simulink library "threeTetCtrllr_ul"  (R2018b)
settings: Solver=VariableStepAuto  StartTime=0.0  StopTime=10.0  RelTol=1e-3
values from neighbouring files (symbols this model uses):
  ctrl = CTR.threeThrCtlr    [threeTetCtrllr_ts.m]
libraries: filteredPIDController_ul x6
settings Model: Creator=Ayaz  LastModifiedBy=asiddiq2

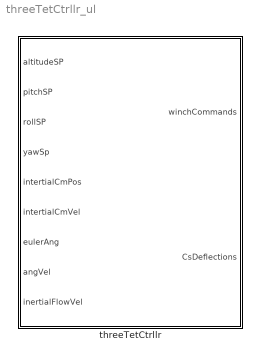
== system threeTetCtrllr_ul ==
  threeTetCtrllr : Subsystem

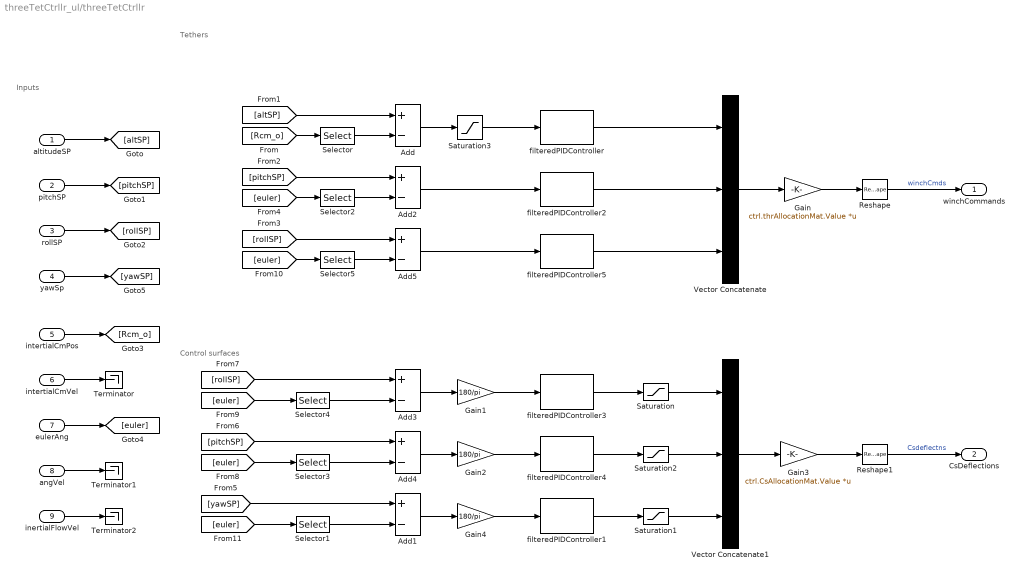
== system threeTetCtrllr_ul/threeTetCtrllr ==
  note: Inputs
  note: Control surfaces
  note: Tethers
  altitudeSP : Inport
  pitchSP : Inport  Port=2
  rollSP : Inport  Port=3
  yawSp : Inport  Port=4
  intertialCmPos : Inport  Port=5
  intertialCmVel : Inport  Port=6
  eulerAng : Inport  Port=7
  angVel : Inport  Port=8
  inertialFlowVel : Inport  Port=9
  Add{,1..5} (6 alike) : Sum  Inputs=+-
  Gain : Gain  Gain=ctrl.thrAllocationMat.Value  Multiplication=Matrix(K*u)
  Gain1 : Gain  Gain=180/pi
  Gain2 : Gain  Gain=180/pi
  Gain3 : Gain  Gain=ctrl.CsAllocationMat.Value  Multiplication=Matrix(K*u)
  Gain4 : Gain  Gain=180/pi
  Reshape : Reshape  OutputDimensionality=Row vector (2-D)
  Reshape1 : Reshape  OutputDimensionality=Column vector (2-D)
  Saturation : Saturate  UpperLimit=ctrl.aileronMaxDef.Value  LowerLimit=-ctrl.aileronMaxDef.Value
  Saturation1 : Saturate  UpperLimit=ctrl.rudderMaxDef.Value  LowerLimit=-ctrl.rudderMaxDef.Value
  Saturation2 : Saturate  UpperLimit=ctrl.elevatorMaxDef.Value  LowerLimit=-ctrl.elevatorMaxDef.Value
  Saturation3 : Saturate  UpperLimit=ctrl.altiErrorSat.Value  LowerLimit=-ctrl.altiErrorSat.Value
  Selector : Selector  NumberOfDimensions=2  InputPortWidth=3  IndexOptions=Index vector (dialog),Index vector (dialog)  Indices=3,1  OutputSizes=1,1
  Selector1 : Selector  NumberOfDimensions=2  InputPortWidth=3  IndexOptions=Index vector (dialog),Index vector (dialog)  Indices=1,1  OutputSizes=1,1
  Selector2 : Selector  NumberOfDimensions=2  InputPortWidth=3  IndexOptions=Index vector (dialog),Index vector (dialog)  Indices=2,1  OutputSizes=1,1
  Selector3 : Selector  NumberOfDimensions=2  InputPortWidth=3  IndexOptions=Index vector (dialog),Index vector (dialog)  Indices=2,1  OutputSizes=1,1
  Selector4 : Selector  NumberOfDimensions=2  InputPortWidth=3  IndexOptions=Index vector (dialog),Index vector (dialog)  Indices=1,1  OutputSizes=1,1
  Selector5 : Selector  NumberOfDimensions=2  InputPortWidth=3  IndexOptions=Index vector (dialog),Index vector (dialog)  Indices=1,1  OutputSizes=1,1
  Terminator : Terminator
  Terminator1 : Terminator
  Terminator2 : Terminator
  Vector Concatenate : Concatenate  NumInputs=3
  Vector Concatenate1 : Concatenate  NumInputs=3
  filteredPIDController : filteredPIDController_ul/filteredPIDController  kp=ctrl.altiTetherKp.Value  ki=ctrl.altiTetherKi.Value  kd=ctrl.altiTetherKd.Value  Value=ctrl.altiTetherTau.Value
  filteredPIDController1 : filteredPIDController_ul/filteredPIDController  kp=ctrl.rudderKp.Value  ki=ctrl.rudderKi.Value  kd=ctrl.rudderKd.Value  Value=ctrl.rudderTau.Value
  filteredPIDController2 : filteredPIDController_ul/filteredPIDController  kp=ctrl.pitchTetherKp.Value  ki=ctrl.pitchTetherKi.Value  kd=ctrl.pitchTetherKd.Value  Value=ctrl.pitchTetherTau.Value
  filteredPIDController3 : filteredPIDController_ul/filteredPIDController  kp=ctrl.aileronKp.Value  ki=ctrl.aileronKi.Value  kd=ctrl.aileronKd.Value  Value=ctrl.aileronTau.Value
  filteredPIDController4 : filteredPIDController_ul/filteredPIDController  kp=ctrl.elevatorKp.Value  ki=ctrl.elevatorKi.Value  kd=ctrl.elevatorKd.Value  Value=ctrl.elevatorTau.Value
  filteredPIDController5 : filteredPIDController_ul/filteredPIDController  kp=ctrl.rollTetherKp.Value  ki=ctrl.rollTetherKi.Value  kd=ctrl.rollTetherKd.Value  Value=ctrl.rollTetherTau.Value
  winchCommands : Outport
  CsDeflections : Outport  Port=2
  wires:
  Add3/1 -> Gain1/1
  Add4/1 -> Gain2/1
  filteredPIDController3/1 -> Saturation/1
  filteredPIDController4/1 -> Saturation2/1
  Selector3/1 -> Add4/2
  [euler] -> Selector3/1
  [pitchSP] -> Add4/1
  Selector4/1 -> Add3/2
  [euler] -> Selector4/1
  Saturation/1 -> Vector Concatenate1/1
  Vector Concatenate1/1 -> Gain3/1
  altitudeSP/1 -> [altSP]
  pitchSP/1 -> [pitchSP]
  rollSP/1 -> [rollSP]
  intertialCmPos/1 -> [Rcm_o]
  eulerAng/1 -> [euler]
  intertialCmVel/1 -> Terminator/1
  angVel/1 -> Terminator1/1
  inertialFlowVel/1 -> Terminator2/1
  Reshape1/1 -> CsDeflections/1  "Csdeflectns"
  Gain1/1 -> filteredPIDController3/1
  Gain2/1 -> filteredPIDController4/1
  [rollSP] -> Add3/1
  Gain4/1 -> filteredPIDController1/1
  [euler] -> Selector1/1
  Selector1/1 -> Add1/2
  [yawSP] -> Add1/1
  filteredPIDController1/1 -> Saturation1/1
  Add1/1 -> Gain4/1
  Selector/1 -> Add/2
  filteredPIDController2/1 -> Vector Concatenate/2
  Saturation3/1 -> filteredPIDController/1
  filteredPIDController5/1 -> Vector Concatenate/3
  Add5/1 -> filteredPIDController5/1
  Add2/1 -> filteredPIDController2/1
  filteredPIDController/1 -> Vector Concatenate/1
  Vector Concatenate/1 -> Gain/1
  Selector5/1 -> Add5/2
  Add/1 -> Saturation3/1
  Selector2/1 -> Add2/2
  Gain/1 -> Reshape/1
  Saturation1/1 -> Vector Concatenate1/3
  Reshape/1 -> winchCommands/1  "winchCmds"
  [altSP] -> Add/1
  [Rcm_o] -> Selector/1
  [pitchSP] -> Add2/1
  [euler] -> Selector2/1
  [rollSP] -> Add5/1
  [euler] -> Selector5/1
  Saturation2/1 -> Vector Concatenate1/2
  Gain3/1 -> Reshape1/1
  yawSp/1 -> [yawSP]
